simulink model "compressor"  (Simulink 7.4)
settings: Solver=ode45  StartTime=0.0  StopTime=300  MaxStep=0.05  RelTol=1e-3
libraries: lib_parallel_comp x1
settings Model: Creator=chkajon  LastModifiedBy=chkajon

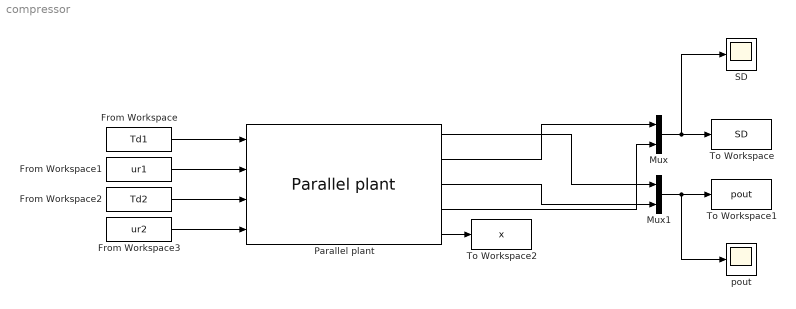
== system compressor ==
  From Workspace : FromWorkspace  VariableName=Td1  SampleTime=0  Interpolate=off  OutputAfterFinalValue=Holding final value
  From Workspace1 : FromWorkspace  VariableName=ur1  SampleTime=0  OutputAfterFinalValue=Holding final value
  From Workspace2 : FromWorkspace  VariableName=Td2  SampleTime=0  OutputAfterFinalValue=Holding final value
  From Workspace3 : FromWorkspace  VariableName=ur2  SampleTime=0  OutputAfterFinalValue=Holding final value
  Mux : Mux  Inputs=2
  Mux1 : Mux  Inputs=2
  Parallel plant : lib_parallel_comp/Parallel plant  SystemSampleTime=-1  x_init_total=xinit  disturbances_on=off  disturbances_symm=off  dist_t_in=0  dist1_in=0  dist2_in=0
  SD : Scope
      settings: YMax=32.5
  To Workspace : ToWorkspace  VariableName=SD  SampleTime=-1  SaveFormat=Structure With Time
  To Workspace1 : ToWorkspace  VariableName=pout  SampleTime=-1  SaveFormat=Structure With Time
  To Workspace2 : ToWorkspace  VariableName=x  SampleTime=-1  SaveFormat=Structure With Time
  pout : Scope
  wires:
  From Workspace/1 -> Parallel plant/1
  From Workspace1/1 -> Parallel plant/2
  From Workspace2/1 -> Parallel plant/3
  From Workspace3/1 -> Parallel plant/4
  Mux/1 -> To Workspace/1, SD/1
  Parallel plant/2 -> Mux/1
  Parallel plant/1 -> Mux1/1
  Mux1/1 -> To Workspace1/1, pout/1
  Parallel plant/3 -> Mux1/2
  Parallel plant/4 -> Mux/2
  Parallel plant/5 -> To Workspace2/1
